simulink library "ScienceStimHasomed_Lib"  (Simulink 6.6)
settings Model: Creator=henrik  LastModifiedBy=henrik

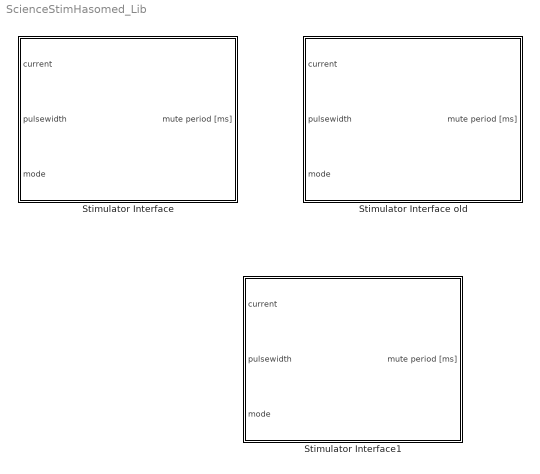
== system ScienceStimHasomed_Lib ==
  Stimulator Interface : Subsystem  mask(Stimulator Interface (RehaStim - Hasomed GmbH)){Ts=0.05, com_port=COM2, channelstim=[1 2], tsone=0, tstwo=5, channellf=[], nfactor=[], outflag=on, dtflag=on}
      mask prompts: Ts "Sample Time:"; com_port "Serial Port:"; channelstim "Channels to be Stimulated:"; tsone "Main Time in ms (only in steps of 0.5 ms):"; tstwo "Group Time in ms (only in steps of 0.5 ms):"; channellf "Low Frequency Channels:"; nfactor "Low Frequency Factor:"; outflag "Enable mute period output"; dtflag "Enable doublets and triplets"
      mask help:
      | Communication to the 8-channel RehaStim Stimulator (HASOMED GmbH) through the serial port.
      |
      | Sample Time:	  The sample time of the block (not neccessarily of the stimulation).
      | Serial Port:	  The serial port connected to the stimulator.
      | Channels:	  An array of channel numbers to be used (e.g. [1 2 5]).
      | Main Time:	  The stimulation period (set this to 0 for external triggering).
      | Group Time:	  The time between pulses in a group (doublet or triplet).
      | Low Freq Ch:	  A sub-set of the channels selected for low frequency.
      | Low Freq Fc:	  Stimulation is only every n times (n=factor).
      mask init:
      | load_system simulink
      | %---------------------------------------------------------------------------
      | % Mute Output
      | % Get the mask parameter values. This is a cell array of strings.
      | maskStr = get_param(gcb,'MaskValues');
      | % The outflag is the 8th mask parameter.
      |     block = 'mute period [ms]';
      |     system_block = [gcb '/' block];
      |     srcblock= 'S-Function';
      |     system_srcblock= [gcb '/' srcblock];
      |     pos=get_param(system_block,'position');
      |     blocktype=get_param(system_block,'blocktype');
      | % Check the value selected 
      | if strcmp(maskStr{8},'on'),
      |     if ~strcmp(blocktype,'Outport')
      |         delete_line(gcb, [srcblock '/1'], [block '/1']);
      |         delete_block(system_block);
      |         add_block('simulink/Sinks/Out1',system_block,'position',pos);
      |         add_line(gcb, [srcblock '/1'], [block '/1']);
      |     end
      | else
      |     if ~strcmp(blocktype,'Terminator')
      |         delete_line(gcb, [srcblock '/1'], [block '/1']);
      |         delete_block(system_block);
      |         add_block('simulink/Sinks/Terminator',system_block,'position',pos);
      |         add_line(gcb, [srcblock '/1'], [block '/1']);
      |     end
      | end
      | %---------------------------------------------------------------------------
      | % Mode input
      | % Get the mask parameter values. This is a cell array of strings.
      | maskStr = get_param(gcb,'MaskValues');
      | % The doublet / triplet flag is the 9th mask parameter.
      |     block = 'mode';
      |     system_block = [gcb '/' block];
      |     sinkblock= 'S-Function';
      |     system_sinkblock= [gcb '/' sinkblock];
      |     pos=get_param(system_block,'position');
      |     blocktype=get_param(system_block,'blocktype');
      | % Check the value selected 
      | if strcmp(maskStr{9},'on'),
      |     if ~strcmp(blocktype,'Inport')
      |         delete_line(gcb, [block '/1'], [sinkblock '/3']);
      |         delete_block(system_block);
      |         add_block('simulink/Sources/In1',system_block,'Port','3','position',pos);
      |         add_line(gcb, [block '/1'], [sinkblock '/3']);
      |     end
      | else % disable mode input, setit to zeros
      |     if ~strcmp(blocktype,'Constant')
      |         delete_line(gcb, [block '/1'], [sinkblock '/3']);
      |         delete_block(system_block);
      |         add_block('simulink/Sources/Constant',system_block,'position',pos);
      |         set_param(system_block,'value','zeros(1,length(channelstim))');
      |         add_line(gcb, [block '/1'], [sinkblock '/3']);
      |     end
      |     % Make sure Group time is large enough if doublet / triplet is off
      |     % It must be at least 1.5 x Number_of_Channels, so we add 0.5 to that
      |     tstwo = 1.5*length(channelstim)+0.5;
      | end
      | 
      | 
      | %---------------------------------------------------------------------------
      | % default minimal Mask Display string
      | MDstr=['image(imread(''RehaStim-background.png''), [0.05 0.25 0.9 0.9]);'...
      |     'port_label(''input'', 1, ''current'');'...
      |     'port_label(''input'', 2, ''pulsewidth'');'...
      |     'text(0.25,0.1,[''Serial Port: COM'' num2str(com_port)],''horizontalAlignment'',''left'',''verticalAlignment'',''bottom'');'...
      |     'text(0.25,0,[''Channels: '' num2str(channelstim)],''horizontalAlignment'',''left'',''verticalAlignment'',''bottom'');'];
      | % get the number of inputs and outputs and add additional labels if needed
      | num_ports=get_param(gcb,'Ports');
      | num_inputs=num_ports(1); num_outputs=num_ports(2);
      | if num_inputs>=3
      |     MDstr=[MDstr 'port_label(''input'', 3, ''mode'');'];
      | end
      | if num_outputs>=1
      |     MDstr=[MDstr 'port_label(''output'', 1, ''mute time [ms]'');'];
      | end
      | set_param(gcb,'MaskDisplay',MDstr)
      mask Help: eval('open(''SciencStimHasomed_Help.html'')')
      mask StyleString: edit,popup(COM1|COM2|COM3|COM4|COM5|COM6|COM7|COM8|COM9|COM10|COM11|COM12|COM13|COM14|COM15|COM16|COM17|COM18|COM19|COM20),edit,edit,edit,edit,edit,checkbox,checkbox
      mask CallbackString:
      | ||||||||% Get the mask parameter values. This is a cell array of strings.
      | maskStr = get_param(gcb,'MaskValues');
      | % The doublet / triplet flag is the 9th mask parameter.
      | % Check the value selected
      | if strcmp(maskStr{9},'on'),
      |     % show associated parameter (Group Time)
      |     set_param(gcb,'MaskVisibilities',{'on';'on';'on';'on';'on';'on';'on';'on';'on'})
      | else
      |     % hide associated parameter (Group Time)
      |     set_param(gcb,'MaskVisibilities',{'on';'on';'on';'on';'off';'on';'on';'on';'on'})
      | end
      mask Display: image(imread('RehaStim-background.png'), [0.05 0.25 0.9 0.9]);port_label('input', 1, 'current');port_label('input', 2, 'pulsewidth');text(0.25,0.1,['Serial Port: COM' num2str(com_port)],'horizontalAlignment','left','verticalAlignment','bottom');text(0.25,0,['Channels: ' num2str(channelstim)],'horizontalAlignment','left','verticalAlignment','bottom');port_label('input', 3, 'mode');port_label('output', 1, 'mute time [ms]');
  Stimulator Interface old : Subsystem  mask(Stimulator Interface (RehaStim - Hasomed GmbH)){Ts=0.05, com_port=COM2, channelstim=[1 2], tsone=0, tstwo=5, channellf=[], nfactor=[]}
      mask prompts: Ts "Sample Time:"; com_port "Serial Port:"; channelstim "Channels to be Stimulated:"; tsone "Main Time in ms (only in steps of 0.5 ms):"; tstwo "Group Time in ms (only in steps of 0.5 ms):"; channellf "Low Frequency Channels:"; nfactor "Low Frequency Factor:"
      mask help:
      | Communication to the 8-channel RehaStim Stimulator (HASOMED GmbH) through the serial port.
      |
      | Sample Time:	  The sample time of the block (not neccessarily of the stimulation).
      | Serial Port:	  The serial port connected to the stimulator.
      | Channels:	  An array of channel numbers to be used (e.g. [1 2 5]).
      | Main Time:	  The stimulation period (set this to 0 for external triggering).
      | Group Time:	  The time between pulses in a group (doublet or triplet).
      | Low Freq Ch:	  A sub-set of the channels selected for low frequency.
      | Low Freq Fc:	  Stimulation is only every n times (n=factor).
      mask Help: eval('open(''SciencStimHasomed_Help.html'')')
      mask StyleString: edit,popup(COM1|COM2|COM3|COM4|COM5|COM6|COM7|COM8|COM9|COM10|COM11|COM12|COM13|COM14|COM15|COM16|COM17|COM18|COM19|COM20),edit,edit,edit,edit,edit
      mask Display:
      | image(imread('RehaStim-background.png'), [0.05 0.25 0.9 0.9]);
      | port_label('input', 1, 'current');
      | port_label('input', 2, 'pulsewidth');
      | port_label('input', 3, 'mode');
      | port_label('output', 1, 'mute period [ms]');
      | text(0.25,0.1,['Serial Port: COM' num2str(com_port)],'horizontalAlignment','left','verticalAlignment','bottom')
      | text(0.25,0,['Channels: ' num2str(channelstim)],'horizontalAlignment','left','verticalAlignment','bottom')
  Stimulator Interface1 : Subsystem  mask(Stimulator Interface (RehaStim - Hasomed GmbH)){Ts=0.05, com_port=COM2, channelstim=[1 2], tsone=0, tstwo=5, channellf=[], nfactor=[], outflag=on, dtflag=on}
      mask prompts: Ts "Sample Time:"; com_port "Serial Port:"; channelstim "Channels to be Stimulated:"; tsone "Main Time in ms (only in steps of 0.5 ms):"; tstwo "Group Time in ms (only in steps of 0.5 ms):"; channellf "Low Frequency Channels:"; nfactor "Low Frequency Factor:"; outflag "Enable mute period output"; dtflag "Enable doublets and triplets"
      mask help:
      | Communication to the 8-channel RehaStim Stimulator (HASOMED GmbH) through the serial port.
      |
      | Sample Time:	  The sample time of the block (not neccessarily of the stimulation).
      | Serial Port:	  The serial port connected to the stimulator.
      | Channels:	  An array of channel numbers to be used (e.g. [1 2 5]).
      | Main Time:	  The stimulation period (set this to 0 for external triggering).
      | Group Time:	  The time between pulses in a group (doublet or triplet).
      | Low Freq Ch:	  A sub-set of the channels selected for low frequency.
      | Low Freq Fc:	  Stimulation is only every n times (n=factor).
      mask init:
      | %---------------------------------------------------------------------------
      | % Mute Output
      | % Get the mask parameter values. This is a cell array of strings.
      | maskStr = get_param(gcb,'MaskValues');
      | % The outflag is the 8th mask parameter.
      |     block = 'mute period [ms]';
      |     system_block = [gcb '/' block];
      |     srcblock= 'S-Function';
      |     system_srcblock= [gcb '/' srcblock];
      |     pos=get_param(system_block,'position');
      |     blocktype=get_param(system_block,'blocktype');
      | % Check the value selected 
      | if strcmp(maskStr{8},'on'),
      |     if ~strcmp(blocktype,'Outport')
      |         delete_line(gcb, [srcblock '/1'], [block '/1']);
      |         delete_block(system_block);
      |         add_block('simulink/Sinks/Out1',system_block,'position',pos);
      |         add_line(gcb, [srcblock '/1'], [block '/1']);
      |     end
      | else
      |     if ~strcmp(blocktype,'Terminator')
      |         delete_line(gcb, [srcblock '/1'], [block '/1']);
      |         delete_block(system_block);
      |         add_block('simulink/Sinks/Terminator',system_block,'position',pos);
      |         add_line(gcb, [srcblock '/1'], [block '/1']);
      |     end
      | end
      | %---------------------------------------------------------------------------
      | % Mode input
      | % Get the mask parameter values. This is a cell array of strings.
      | maskStr = get_param(gcb,'MaskValues');
      | % The doublet / triplet flag is the 9th mask parameter.
      |     block = 'mode';
      |     system_block = [gcb '/' block];
      |     sinkblock= 'S-Function';
      |     system_sinkblock= [gcb '/' sinkblock];
      |     pos=get_param(system_block,'position');
      |     blocktype=get_param(system_block,'blocktype');
      | % Check the value selected 
      | if strcmp(maskStr{9},'on'),
      |     if ~strcmp(blocktype,'Inport')
      |         delete_line(gcb, [block '/1'], [sinkblock '/3']);
      |         delete_block(system_block);
      |         add_block('simulink/Sources/In1',system_block,'Port','3','position',pos);
      |         add_line(gcb, [block '/1'], [sinkblock '/3']);
      |     end
      | else % disable mode input, setit to zeros
      |     if ~strcmp(blocktype,'Constant')
      |         delete_line(gcb, [block '/1'], [sinkblock '/3']);
      |         delete_block(system_block);
      |          add_block('simulink/Sources/Constant',system_block,'position',pos);
      |         if exist('channelstim')
      |             channelstim=[];
      |         end
      |         set_param(system_block,'value','zeros(1,length(channelstim))');
      |         add_line(gcb, [block '/1'], [sinkblock '/3']);
      |     end
      | end
      | 
      | %---------------------------------------------------------------------------
      | % default minimal Mask Display string
      | MDstr=['image(imread(''RehaStim-background.png''), [0.05 0.25 0.9 0.9]);'...
      |     'port_label(''input'', 1, ''current'');'...
      |     'port_label(''input'', 2, ''pulsewidth'');'...
      |     'text(0.25,0.1,[''Serial Port: COM'' num2str(com_port)],''horizontalAlignment'',''left'',''verticalAlignment'',''bottom'');'...
      |     'text(0.25,0,[''Channels: '' num2str(channelstim)],''horizontalAlignment'',''left'',''verticalAlignment'',''bottom'');'];
      | % get the number of inputs and outputs and add additional labels if needed
      | num_ports=get_param(gcb,'Ports');
      | num_inputs=num_ports(1); num_outputs=num_ports(2);
      | if num_inputs>=3
      |     MDstr=[MDstr 'port_label(''input'', 3, ''mode'');'];
      | end
      | if num_outputs>=1
      |     MDstr=[MDstr 'port_label(''output'', 1, ''mute time [ms]'');'];
      | end
      | set_param(gcb,'MaskDisplay',MDstr)
      mask Help: eval('open(''SciencStimHasomed_Help.html'')')
      mask StyleString: edit,popup(COM1|COM2|COM3|COM4|COM5|COM6|COM7|COM8|COM9|COM10|COM11|COM12|COM13|COM14|COM15|COM16|COM17|COM18|COM19|COM20),edit,edit,edit,edit,edit,checkbox,checkbox
      mask CallbackString:
      | ||||||||% Get the mask parameter values. This is a cell array of strings.
      | maskStr = get_param(gcb,'MaskValues');
      | % The doublet / triplet flag is the 9th mask parameter.
      | % Check the value selected
      | if strcmp(maskStr{9},'on'),
      |     % show associated parameter (Group Time)
      |     set_param(gcb,'MaskVisibilities',{'on';'on';'on';'on';'on';'on';'on';'on';'on'})
      | else
      |     % hide associated parameter (Group Time)
      |     set_param(gcb,'MaskVisibilities',{'on';'on';'on';'on';'off';'on';'on';'on';'on'})
      |     % Make sure Group time is large enough if doublet / triplet is off
      |     % It must be at least 1.5 x Number_of_Channels, so we add 0.5 to that
      |     tstwo = 1.5*length(channelstim)+0.5;
      | end
      mask Display: image(imread('RehaStim-background.png'), [0.05 0.25 0.9 0.9]);port_label('input', 1, 'current');port_label('input', 2, 'pulsewidth');text(0.25,0.1,['Serial Port: COM' num2str(com_port)],'horizontalAlignment','left','verticalAlignment','bottom');text(0.25,0,['Channels: ' num2str(channelstim)],'horizontalAlignment','left','verticalAlignment','bottom');port_label('input', 3, 'mode');port_label('output', 1, 'mute time [ms]');

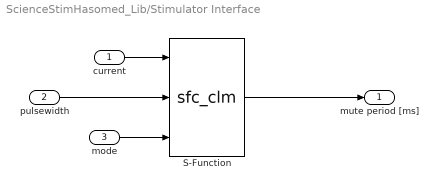
== system ScienceStimHasomed_Lib/Stimulator Interface ==
  current : Inport
  pulsewidth : Inport  Port=2
  mode : Inport  Port=3
  S-Function : S-Function  FunctionName=sfc_clm  Parameters=Ts,com_port,channelstim,tsone,tstwo,0,channellf,nfactor
  mute period [ms] : Outport
  wires:
  current/1 -> S-Function/1
  pulsewidth/1 -> S-Function/2
  S-Function/1 -> mute period [ms]/1
  mode/1 -> S-Function/3

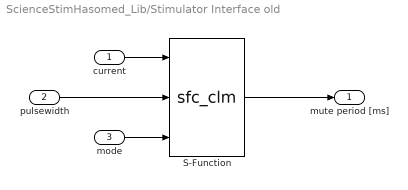
== system ScienceStimHasomed_Lib/Stimulator Interface old ==
  current : Inport
  pulsewidth : Inport  Port=2
  mode : Inport  Port=3
  S-Function : S-Function  FunctionName=sfc_clm  Parameters=Ts,com_port,channelstim,tsone,tstwo,0,channellf,nfactor
  mute period [ms] : Outport
  wires:
  S-Function/1 -> mute period [ms]/1
  mode/1 -> S-Function/3
  pulsewidth/1 -> S-Function/2
  current/1 -> S-Function/1

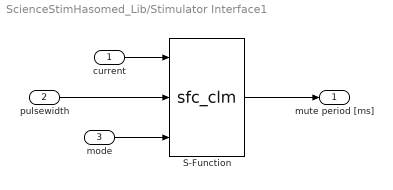
== system ScienceStimHasomed_Lib/Stimulator Interface1 ==
  current : Inport
  pulsewidth : Inport  Port=2
  mode : Inport  Port=3
  S-Function : S-Function  FunctionName=sfc_clm  Parameters=Ts,com_port,channelstim,tsone,tstwo,0,channellf,nfactor
  mute period [ms] : Outport
  wires:
  mode/1 -> S-Function/3
  S-Function/1 -> mute period [ms]/1
  pulsewidth/1 -> S-Function/2
  current/1 -> S-Function/1
